simulink model "Test_CP"  (R2026a)
settings: configuration reference "testConfig" (kept outside this file)
model workspace (MAT data in the model file):
  p1 = Simulink.Parameter
  p1.Value = [1  2; 3  4]
  p1.Complexity = 'real'
  p1.Dimensions = [2 2]
  p1.CoderInfo.StorageClass = 'SimulinkGlobal'
  p1.DataType = 'int8'
  ps = Simulink.Parameter
  ps.Value.p1 = 1
  ps.Value.psi.psi1 = 1
  ps.Complexity = 'real'
  ps.Dimensions = [1 1]
  ps.CoderInfo.StorageClass = 'SimulinkGlobal'
  ps.DataType = 'struct'
  ps_p1 = Simulink.Parameter
  ps_p1.Value = 1
  ps_p1.Complexity = 'real'
  ps_p1.Dimensions = [1 1]
  ps_p1.CoderInfo.StorageClass = 'SimulinkGlobal'
  ps_p1.DataType = 'int8'
values from neighbouring files (symbols this model uses):
  ddParam = 2.0    [MyParams.sldd]
settings Model: DataDictionary=MyParams.sldd  ParameterArgumentNames=p1,ps,ps_p1  Creator=toma  LastModifiedBy=toma
settings ConfigSetRef: SourceName=testConfig

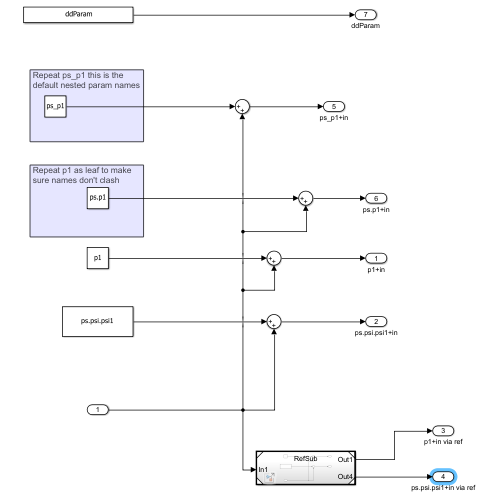
[thumbnail: Simulink's stored preview of the top-level diagram]
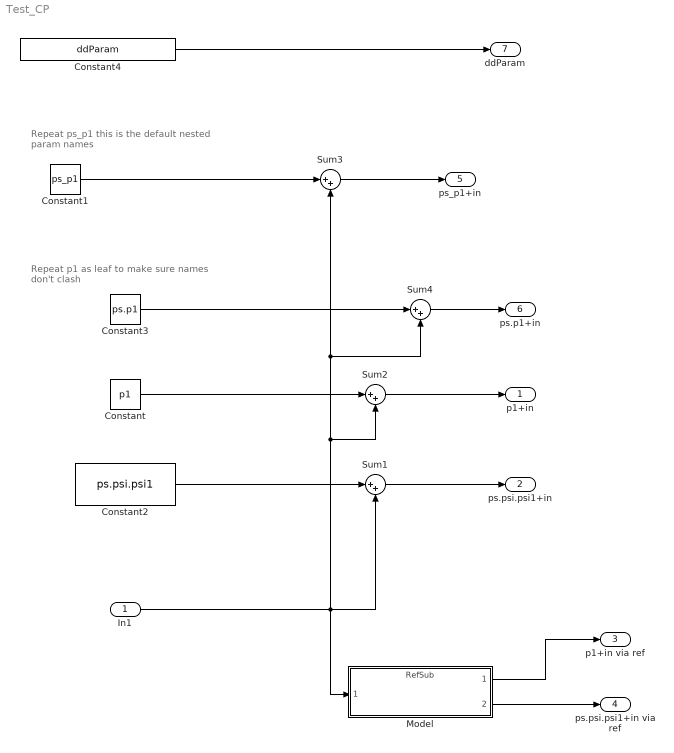
== system Test_CP ==
  note: Repeat p1 as leaf to make
      | sure names don't clash
  note: Repeat ps_p1 this is the
      | default nested param names
  In1 : Inport  OutDataTypeStr=double  PortDimensions=1  SampleTime=[0.20000000000000001,0]
  Constant : Constant  Value=p1
  Constant1 : Constant  Value=ps_p1
  Constant2 : Constant  Value=ps.psi.psi1
  Constant3 : Constant  Value=ps.p1
  Constant4 : Constant  Value=ddParam
  Model : ModelReference  ModelNameDialog=RefSub.slx  UsingDefaultArgumentValue=0,0  SimulationMode=Normal  ModelReferenceVersion=13.0
  Sum{1..4} (4 alike) : Sum  Inputs=|++
  p1+in : Outport  OutDataTypeStr=double  PortDimensions=[2 2]  SampleTime=[0.20000000000000001,0]
  ps.psi.psi1+in : Outport  Port=2  OutDataTypeStr=double  PortDimensions=1  SampleTime=[0.20000000000000001,0]
  p1+in via ref : Outport  Port=3  OutDataTypeStr=double  PortDimensions=[2 2]  SampleTime=[0.20000000000000001,0]
  ps.psi.psi1+in via ref : Outport  Port=4  OutDataTypeStr=double  PortDimensions=1  SampleTime=[0.20000000000000001,0]
  ps_p1+in : Outport  Port=5
  ps.p1+in : Outport  Port=6
  ddParam : Outport  Port=7
  wires:
  Sum1/1 -> ps.psi.psi1+in/1
  In1/1 -> Sum2/2, Sum3/2, Sum4/2, Model/1, Sum1/2
  Constant/1 -> Sum2/1
  Constant2/1 -> Sum1/1
  Sum2/1 -> p1+in/1
  Model/1 -> p1+in via ref/1
  Model/2 -> ps.psi.psi1+in via ref/1
  Sum3/1 -> ps_p1+in/1
  Constant1/1 -> Sum3/1
  Constant3/1 -> Sum4/1
  Sum4/1 -> ps.p1+in/1
  Constant4/1 -> ddParam/1
